simulink model "model_reg"  (R2022b)
settings: Solver=ode3  StartTime=0.0  StopTime=Tmdl  FixedStep=T/1000  RelTol=1e-3
values from neighbouring files (symbols this model uses):
  K1 = 85    [data.mat]
  K2 = 70    [data.mat]
  K3 = 0.02    [data.mat]
  T1 = 0.09    [data.mat]
  T2 = 0.1    [data.mat]
undefined symbols (not defined in the file or in its folder): K
settings Model: Creator=R1505-We2-2-Stud  LastModifiedBy=R1505-We2-2-Stud

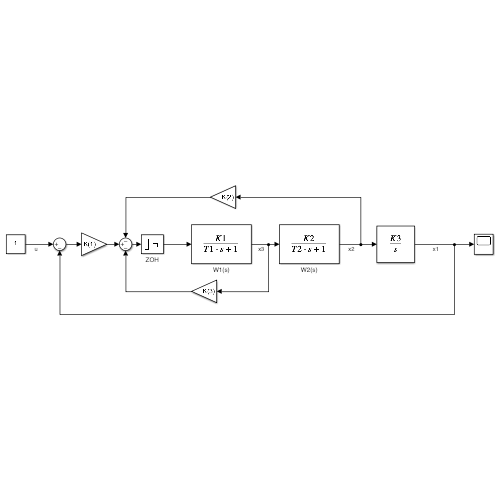
[thumbnail: Simulink's stored preview of the top-level diagram]
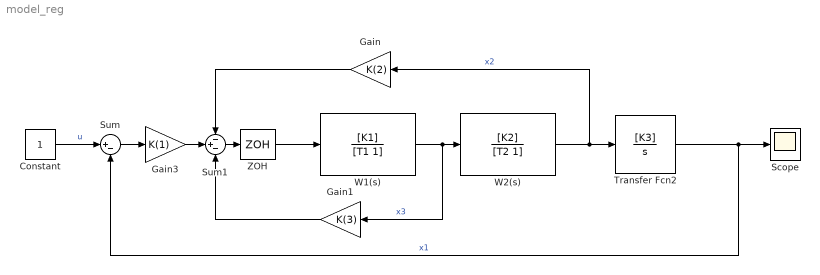
== system model_reg ==
  Constant : Constant
  Gain : Gain  Gain=K(2)
  Gain1 : Gain  Gain=K(3)
  Gain3 : Gain  Gain=K(1)
  Scope : Scope
  Sum : Sum  Inputs=|+-
  Sum1 : Sum  Inputs=-+-
  Transfer Fcn2 : TransferFcn  Numerator=[K3]  Denominator=[1 0]
  W1(s) : TransferFcn  Numerator=[K1]  Denominator=[T1 1]
  W2(s) : TransferFcn  Numerator=[K2]  Denominator=[T2 1]
  ZOH : ZeroOrderHold  SampleTime=-1
  wires:
  W1(s)/1 -> Gain1/1, W2(s)/1  "x3"
  W2(s)/1 -> Gain/1, Transfer Fcn2/1  "x2"
  ZOH/1 -> W1(s)/1
  Transfer Fcn2/1 -> Scope/1, Sum/2  "x1"
  Constant/1 -> Sum/1  "u"
  Gain3/1 -> Sum1/2
  Sum/1 -> Gain3/1
  Sum1/1 -> ZOH/1
  Gain/1 -> Sum1/1
  Gain1/1 -> Sum1/3
